simulink model "servom"  (R2022b)
settings: Solver=VariableStepAuto  StartTime=0.0  StopTime=10.0  RelTol=1e-3
undefined symbols (not defined in the file or in its folder): magnitude
settings Model: Creator=antoine  LastModifiedBy=kbada

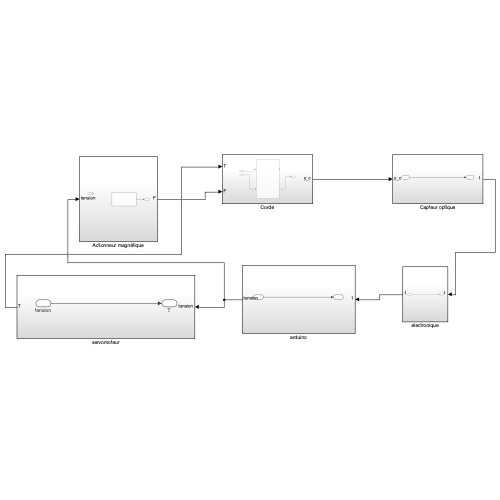
[thumbnail: Simulink's stored preview of the top-level diagram]
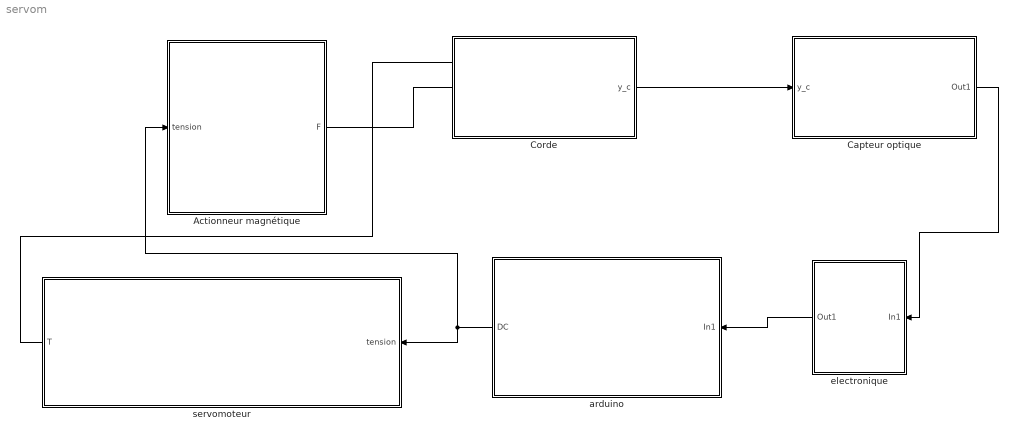
== system servom ==
  Actionneur magnétique : Subsystem
  Capteur optique : Subsystem
  Corde : Subsystem
  arduino : Subsystem
  electronique : Subsystem
  servomoteur : Subsystem
  wires:
  Actionneur magnétique/1(F) -> ?
  Corde/1(y_c) -> Capteur optique/1(y_c)
  Capteur optique/1(Out1) -> electronique/1(In1)
  arduino/1(DC) -> servomoteur/1(tension), Actionneur magnétique/1(tension)
  servomoteur/1(T) -> ?
  electronique/1(Out1) -> arduino/1(In1)

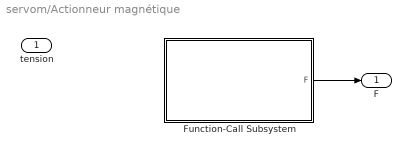
== system servom/Actionneur magnétique ==
  tension : Inport
  Function-Call Subsystem : Subsystem  TreatAsAtomicUnit=on
  F : Outport
  wires:
  Function-Call Subsystem/1(F) -> F/1

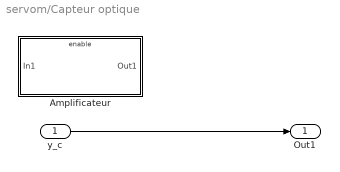
== system servom/Capteur optique ==
  y_c : Inport
  Amplificateur : Subsystem  TreatAsAtomicUnit=on
  Out1 : Outport
  wires:
  y_c/1 -> Out1/1

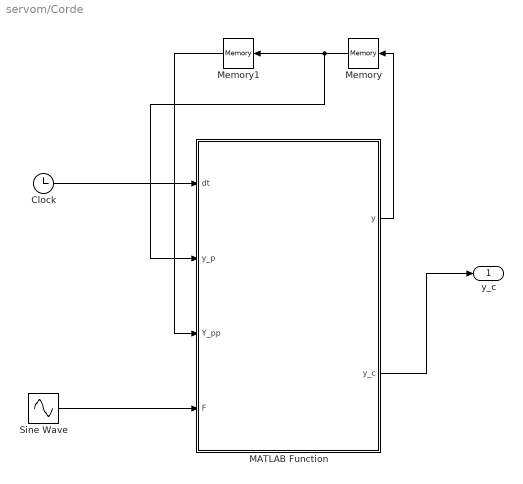
== system servom/Corde ==
  Clock : Clock
  MATLAB Function : MATLAB Function  TreatAsAtomicUnit=on
  Memory : Memory
  Memory1 : Memory
  Sine Wave : Sin  SampleTime=0
  y_c : Outport
  wires:
  Sine Wave/1 -> MATLAB Function/4(F)
  Clock/1 -> MATLAB Function/1(dt)
  MATLAB Function/2(y_c) -> y_c/1
  Memory/1 -> MATLAB Function/2(y_p), Memory1/1
  MATLAB Function/1(y) -> Memory/1
  Memory1/1 -> MATLAB Function/3(Y_pp)

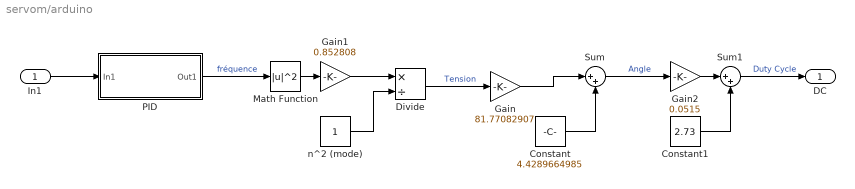
== system servom/arduino ==
  In1 : Inport
  Constant : Constant  Value=4.4289664985
  Constant1 : Constant  Value=2.73
  Divide : Product  Inputs=*/
  Gain : Gain  Gain=81.77082907
  Gain1 : Gain  Gain=0.852808
  Gain2 : Gain  Gain=0.0515
  Math Function : Math  Operator=magnitude^2
  PID : Subsystem
  Sum : Sum  Inputs=|++
  Sum1 : Sum  Inputs=|++
  n^2 (mode) : Constant
  DC : Outport
  wires:
  In1/1 -> PID/1(In1)
  Gain/1 -> Sum/1
  Constant/1 -> Sum/2
  PID/1(Out1) -> Math Function/1  "fréquence"
  Math Function/1 -> Gain1/1
  Divide/1 -> Gain/1  "Tension"
  Sum/1 -> Gain2/1  "Angle"
  Constant1/1 -> Sum1/2
  Gain2/1 -> Sum1/1
  Gain1/1 -> Divide/1
  n^2 (mode)/1 -> Divide/2
  Sum1/1 -> DC/1  "Duty Cycle"

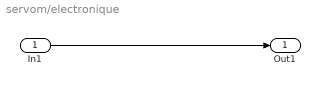
== system servom/electronique ==
  In1 : Inport
  Out1 : Outport
  wires:
  In1/1 -> Out1/1

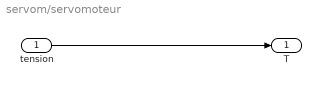
== system servom/servomoteur ==
  tension : Inport
  T : Outport
  wires:
  tension/1 -> T/1

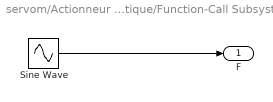
== system servom/Actionneur magnétique/Function-Call Subsystem ==
  Sine Wave : Sin  Frequency=80*2*3.1416  SampleTime=0
  F : Outport
  wires:
  Sine Wave/1 -> F/1

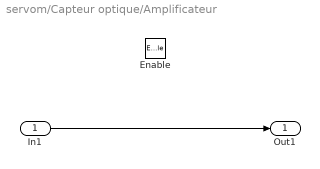
== system servom/Capteur optique/Amplificateur ==
  In1 : Inport
  Enable : EnablePort
  Out1 : Outport
  wires:
  In1/1 -> Out1/1

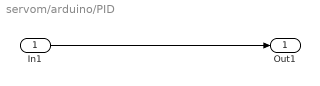
== system servom/arduino/PID ==
  In1 : Inport
  Out1 : Outport
  wires:
  In1/1 -> Out1/1

== matlab function servom/Corde/MATLAB Function ==
  data: y output; dt input; y_p input; Y_pp input; y_c output; F input
function [y,y_c] = corde(dt, y_p, Y_pp,F)

f_1 = 100;
b = 3.26 *10^(-3);
mu = 7.68 * 10^(-3);
masse = 0.004405; %[kg]
Longueur = 0.44; %[m]
Tension = f_1^2 * 4 *Longueur^2 * mu;
n = 11; % découper la corde en n morceaux
p_actionneur = floorDiv(n*3,4);
p_capteur = floorDiv(n,4);
y = zeros(1,n);
f = zeros(1,n);
f(p_actionneur) = F;
beta = 1/2 *b*dt;

for i = 2:(n-1)
    pos = y_p(i+1) - 2*y_p(i) + y_p(i-1);
    y(i) = ((1 + beta)^(-1)) * ((beta-1)*y_pp(i) +2*y_p(i) + c^2 *(pos) + dt^2 * f(i));
end




end
